simulink model "SC228_TrackedASModelUnitTest"  (R2018b)
settings: Solver=VariableStepAuto  StartTime=0.0  StopTime=10.0  RelTol=1e-3
undefined symbols (not defined in the file or in its folder): ac1dyn_alt0_ft, ac1dyn_con, ac1dyn_lat0_rad, ac1dyn_lon0_rad, ac2dyn_alt0_ft, ac2dyn_con, ac2dyn_lat0_rad, ac2dyn_lon0_rad, ddh_ftps2, dh_ftps, dv_ftps2, e_ft, Edot_ftps, h_ft, hdot_ftps, latLonAltState, n_ft, Ndot_ftps, p_radps, phi_rad, phidot_radps, psi_rad, psidot_radps, q_radps, r_radps, theta_rad, thetadot_radps, uas_tcas_trckd_altQuant_ft, uas_tcas_trckd_bearing_Breakpoints_deg, uas_tcas_trckd_bearing_Max_deg, uas_tcas_trckd_bearing_Sigma_deg, uas_tcas_trckd_dt_s, uas_tcas_trckd_FOR_elev_max_deg, uas_tcas_trckd_FOR_elev_min_deg, uas_tcas_trckd_probDetect, uas_tcas_trckd_psi_bias_ft, uas_tcas_trckd_psi_stddev_ft, uas_tcas_trckd_psidot_bias_radps, uas_tcas_trckd_psidot_stddev_ftps, uas_tcas_trckd_randProbSeed, uas_tcas_trckd_reported_errorCovRBA, uas_tcas_trckd_rng_bias_ft, uas_tcas_trckd_rng_random_stddev_ft, uas_tcas_trckd_seed1, uas_tcas_trckd_seed2, uas_tcas_trckd_seed3, uas_tcas_trckd_seed4, uas_tcas_trckd_sns_max_front_range_ft, uas_tcas_trckd_sns_max_range_ft, uas_tcas_trckd_sns_max_rear_range_ft, uas_tcas_trckd_sns_max_side_range_ft, uas_tcas_trckd_tauThreshold_sec, uas_tcas_trckd_updateRate_sec, v_ftps, vdot_fpss
libraries: simulink x20, dspmtrx3 x1
(part 2 of 2)

== system SC228_TrackedASModelUnitTest/AC2 - Track Following/Follow Trajectory/Set State ==
  x : Inport
  Bus Assignment : BusAssignment  AssignedSignals=v_ftps,n_ft,e_ft,h_ft,psi_rad,theta_rad,phi_rad,dv_ftps2,dh_ftps,ddh_ftps2
  Demux : Demux  Outputs=10
  Null AircraftState : Subsystem
  State : Outport
  wires:
  Demux/10 -> Bus Assignment/11
  Demux/9 -> Bus Assignment/10
  Bus Assignment/1 -> State/1
  Null AircraftState/1(State) -> Bus Assignment/1
  Demux/7 -> Bus Assignment/8  "phi"
  x/1 -> Demux/1
  Demux/6 -> Bus Assignment/7  "theta"
  Demux/5 -> Bus Assignment/6  "psi"
  Demux/4 -> Bus Assignment/5  "h"
  Demux/3 -> Bus Assignment/4  "E"
  Demux/2 -> Bus Assignment/3  "N"
  Demux/1 -> Bus Assignment/2  "v"
  Demux/8 -> Bus Assignment/9  "a"

== system SC228_TrackedASModelUnitTest/SC-228 Sensor Model: Active Surveillance (Tracked)/Add Errors/Colored Noise1 ==
  Add : Sum  Inputs=+++
  Add1 : Sum
  Constant : Constant  Value=false
  Constant1 : Constant  Value=0
  Gain : Gain  Gain=exp(-dt(1)/tau)
  Gain1 : Gain  Gain=sig*sqrt(1-(exp(-dt(1)/tau))*(exp(-dt(1)/tau)))
  Gain2 : Gain  Gain=sig
  IsInitial : Memory  InitialCondition=true  InheritSampleTime=on
  Memory : Memory  InheritSampleTime=on
  Random Number : RandomNumber  Seed=seed  SampleTime=dt_s
  Switch : Switch  Criteria=u2 ~= 0
  bias : Constant  Value=bias
  noisy : Outport
  wires:
  Gain1/1 -> Add1/2  "uncorrelated error"
  Switch/1 -> Memory/1, Add/3  "colored random error"
  bias/1 -> Add/2  "fixed bias"
  Random Number/1 -> Gain2/1, Gain1/1
  Gain/1 -> Add1/1  "correlated error"
  Add/1 -> noisy/1  "noisy state parameter"
  Memory/1 -> Gain/1
  Constant/1 -> IsInitial/1
  IsInitial/1 -> Switch/2
  Add1/1 -> Switch/3  "colored random error"
  Gain2/1 -> Switch/1
  Constant1/1 -> Add/1

== system SC228_TrackedASModelUnitTest/SC-228 Sensor Model: Active Surveillance (Tracked)/Add Errors/Colored Noise2 ==
  Add : Sum  Inputs=+++
  Add1 : Sum
  Constant : Constant  Value=false
  Constant1 : Constant  Value=0
  Gain : Gain  Gain=exp(-dt(1)/tau)
  Gain1 : Gain  Gain=sig*sqrt(1-(exp(-dt(1)/tau))*(exp(-dt(1)/tau)))
  Gain2 : Gain  Gain=sig
  IsInitial : Memory  InitialCondition=true  InheritSampleTime=on
  Memory : Memory  InheritSampleTime=on
  Random Number : RandomNumber  Seed=seed  SampleTime=dt_s
  Switch : Switch  Criteria=u2 ~= 0
  bias : Constant  Value=bias
  noisy : Outport
  wires:
  Gain1/1 -> Add1/2  "uncorrelated error"
  Switch/1 -> Memory/1, Add/3  "colored random error"
  bias/1 -> Add/2  "fixed bias"
  Random Number/1 -> Gain2/1, Gain1/1
  Gain/1 -> Add1/1  "correlated error"
  Add/1 -> noisy/1  "noisy state parameter"
  Memory/1 -> Gain/1
  Constant/1 -> IsInitial/1
  IsInitial/1 -> Switch/2
  Add1/1 -> Switch/3  "colored random error"
  Gain2/1 -> Switch/1
  Constant1/1 -> Add/1

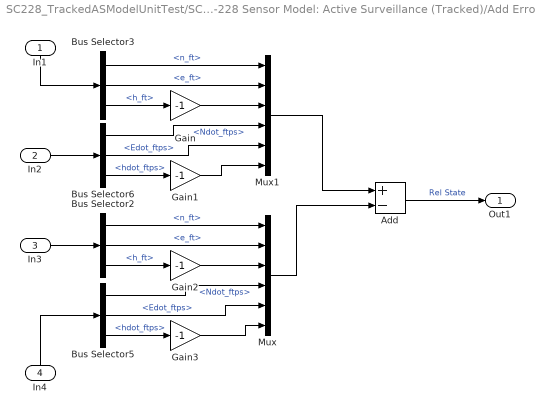
== system SC228_TrackedASModelUnitTest/SC-228 Sensor Model: Active Surveillance (Tracked)/Add Errors/Compute Relative State ==
  In1 : Inport
  In2 : Inport  Port=2
  In3 : Inport  Port=3
  In4 : Inport  Port=4
  Add : Sum  Inputs=+-
  Bus Selector2 : BusSelector  OutputSignals=n_ft,e_ft,h_ft
  Bus Selector3 : BusSelector  OutputSignals=n_ft,e_ft,h_ft
  Bus Selector5 : BusSelector  OutputSignals=Ndot_ftps,Edot_ftps,hdot_ftps
  Bus Selector6 : BusSelector  OutputSignals=Ndot_ftps,Edot_ftps,hdot_ftps
  Gain{,1..3} (4 alike) : Gain  Gain=-1
  Mux : Mux  Inputs=6
  Mux1 : Mux  Inputs=6
  Out1 : Outport
  wires:
  Bus Selector5/1 -> Mux/4  "<Ndot_ftps>"
  Bus Selector5/2 -> Mux/5  "<Edot_ftps>"
  In2/1 -> Bus Selector6/1
  Bus Selector3/3 -> Gain/1  "<h_ft>"
  Bus Selector2/3 -> Gain2/1  "<h_ft>"
  Bus Selector5/3 -> Gain3/1  "<hdot_ftps>"
  Bus Selector2/2 -> Mux/2  "<e_ft>"
  Mux1/1 -> Add/1
  In4/1 -> Bus Selector5/1
  In3/1 -> Bus Selector2/1
  Add/1 -> Out1/1  "Rel State"
  Mux/1 -> Add/2
  Bus Selector2/1 -> Mux/1  "<n_ft>"
  Bus Selector3/1 -> Mux1/1  "<n_ft>"
  Bus Selector3/2 -> Mux1/2  "<e_ft>"
  In1/1 -> Bus Selector3/1
  Bus Selector6/3 -> Gain1/1  "<hdot_ftps>"
  Bus Selector6/1 -> Mux1/4  "<Ndot_ftps>"
  Bus Selector6/2 -> Mux1/5  "<Edot_ftps>"
  Gain/1 -> Mux1/3
  Gain1/1 -> Mux1/6
  Gain2/1 -> Mux/3
  Gain3/1 -> Mux/6

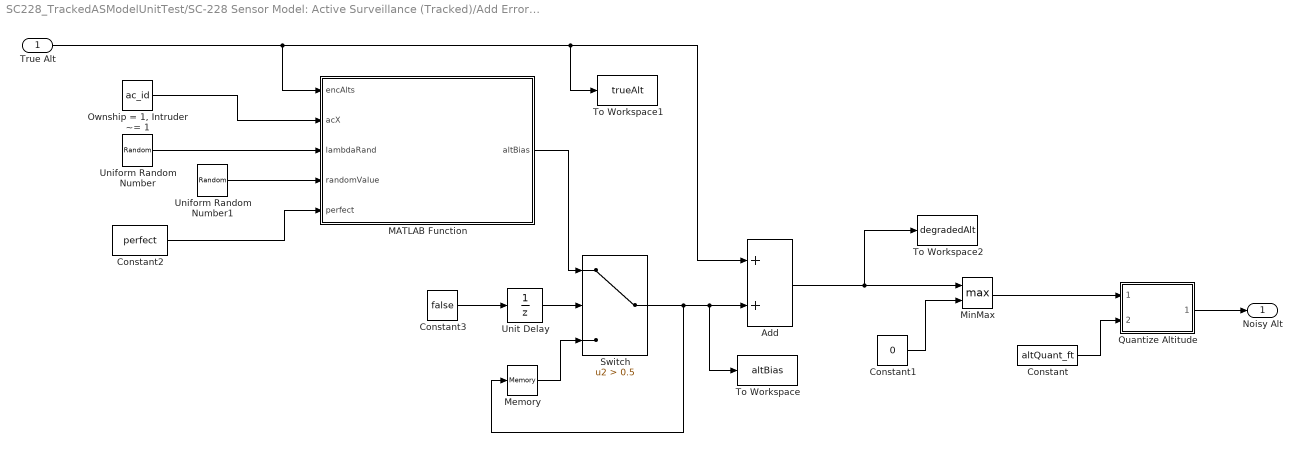
== system SC228_TrackedASModelUnitTest/SC-228 Sensor Model: Active Surveillance (Tracked)/Add Errors/TSAA Altitude Error Model ==
  True Alt : Inport
  Add : Sum
  Constant : Constant  Value=altQuant_ft
  Constant1 : Constant  Value=0
  Constant2 : Constant  Value=perfect
  Constant3 : Constant  Value=false
  MATLAB Function : MATLAB Function  TreatAsAtomicUnit=on
  Memory : Memory
  MinMax : MinMax  Function=max  Inputs=2
  "Ownship = 1, Intruder ~= 1" : Constant  Value=ac_id
  Quantize Altitude : Subsystem
  Switch : Switch  Criteria=u2 > Threshold  Threshold=0.5
  To Workspace : ToWorkspace  VariableName=altBias  SaveFormat=Timeseries  SampleTime=-1
  To Workspace1 : ToWorkspace  VariableName=trueAlt  SaveFormat=Timeseries  SampleTime=-1
  To Workspace2 : ToWorkspace  VariableName=degradedAlt  SaveFormat=Timeseries  SampleTime=-1
  Uniform Random Number : UniformRandomNumber  Minimum=0  Seed=lambdaSeed  SampleTime=dt_s
  Uniform Random Number1 : UniformRandomNumber  Minimum=0  Seed=randomSeed  SampleTime=dt_s
  Unit Delay : UnitDelay  InitialCondition=true  SampleTime=-1
  Noisy Alt : Outport
  wires:
  Constant2/1 -> MATLAB Function/5(perfect)
  Quantize Altitude/1(Quantized Alt) -> Noisy Alt/1
  MinMax/1 -> Quantize Altitude/1(Altitude)
  Constant1/1 -> MinMax/2
  "Ownship = 1, Intruder ~= 1"/1 -> MATLAB Function/2(acX)
  True Alt/1 -> To Workspace1/1, Add/1, MATLAB Function/1(encAlts)
  Uniform Random Number/1 -> MATLAB Function/3(lambdaRand)
  Uniform Random Number1/1 -> MATLAB Function/4(randomValue)
  MATLAB Function/1(altBias) -> Switch/1
  Constant3/1 -> Unit Delay/1
  Unit Delay/1 -> Switch/2
  Switch/1 -> To Workspace/1, Add/2, Memory/1
  Memory/1 -> Switch/3
  Constant/1 -> Quantize Altitude/2(Quant_level)
  Add/1 -> To Workspace2/1, MinMax/1

== system SC228_TrackedASModelUnitTest/SC-228 Sensor Model: Active Surveillance (Tracked)/Add Errors/White Noise ==
  bearing : Inport
  MATLAB Function : MATLAB Function  TreatAsAtomicUnit=on
  Random Number : RandomNumber  Seed=seed_bearing  SampleTime=dt_s
  Terminator : Terminator
  To Workspace : ToWorkspace  VariableName=psi  SaveFormat=Timeseries  SampleTime=-1
  "noisy " : Outport
  psiSigma : Outport  Port=2
  wires:
  MATLAB Function/1(sigma) -> psiSigma/1
  MATLAB Function/2(max) -> Terminator/1
  bearing/1 -> [psi]
  [psi] -> To Workspace/1, "noisy "/1, MATLAB Function/1(psi)

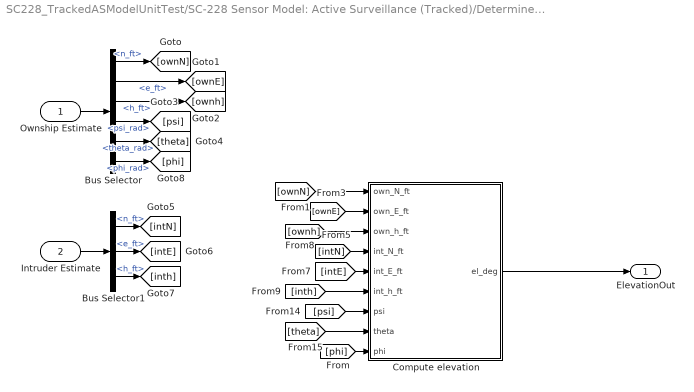
== system SC228_TrackedASModelUnitTest/SC-228 Sensor Model: Active Surveillance (Tracked)/Determine Track Validity/Compute Elevation ==
  Ownship Estimate : Inport
  Intruder Estimate : Inport  Port=2
  Bus Selector : BusSelector  OutputSignals=n_ft,e_ft,h_ft,psi_rad,theta_rad,phi_rad
  Bus Selector1 : BusSelector  OutputSignals=n_ft,e_ft,h_ft
  Compute elevation : MATLAB Function  TreatAsAtomicUnit=on
  ElevationOut : Outport
  wires:
  Ownship Estimate/1 -> Bus Selector/1
  Compute elevation/1(el_deg) -> ElevationOut/1
  Intruder Estimate/1 -> Bus Selector1/1
  Bus Selector/1 -> [ownN]  "<n_ft>"
  Bus Selector/2 -> [ownE]  "<e_ft>"
  Bus Selector/3 -> [ownh]  "<h_ft>"
  Bus Selector/4 -> [psi]  "<psi_rad>"
  Bus Selector/5 -> [theta]  "<theta_rad>"
  Bus Selector1/1 -> [intN]  "<n_ft>"
  Bus Selector1/2 -> [intE]  "<e_ft>"
  Bus Selector1/3 -> [inth]  "<h_ft>"
  [ownN] -> Compute elevation/1(own_N_ft)
  [ownE] -> Compute elevation/2(own_E_ft)
  [intN] -> Compute elevation/4(int_N_ft)
  [intE] -> Compute elevation/5(int_E_ft)
  [ownh] -> Compute elevation/3(own_h_ft)
  [inth] -> Compute elevation/6(int_h_ft)
  [psi] -> Compute elevation/7(psi)
  [theta] -> Compute elevation/8(theta)
  Bus Selector/6 -> [phi]  "<phi_rad>"
  [phi] -> Compute elevation/9(phi)

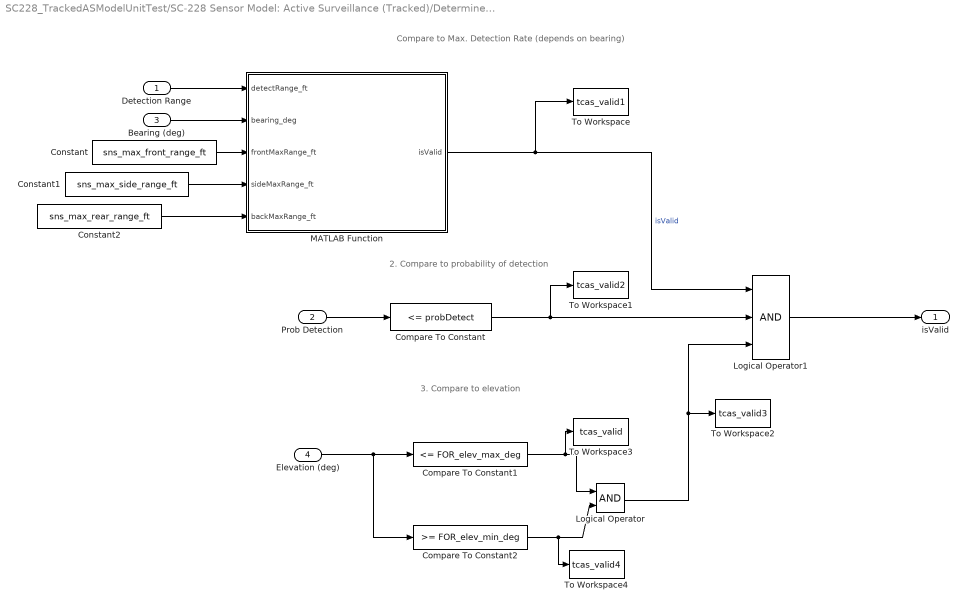
== system SC228_TrackedASModelUnitTest/SC-228 Sensor Model: Active Surveillance (Tracked)/Determine Track Validity/Determine Validity  ==
  note: 3. Compare to elevation
  note: 2. Compare to probability of detection
  note: Compare to Max. Detection Rate (depends on bearing)
  Detection Range : Inport
  Prob Detection : Inport  Port=2
  Bearing (deg) : Inport  Port=3
  Elevation (deg) : Inport  Port=4
  Compare To Constant : simulink/Logic and Bit Operations/Compare To Constant  relop=<=  const=probDetect  OutDataTypeStr=boolean
  Compare To Constant1 : simulink/Logic and Bit Operations/Compare To Constant  relop=<=  const=FOR_elev_max_deg  OutDataTypeStr=boolean
  Compare To Constant2 : simulink/Logic and Bit Operations/Compare To Constant  relop=>=  const=FOR_elev_min_deg  OutDataTypeStr=boolean
  Constant : Constant  Value=sns_max_front_range_ft
  Constant1 : Constant  Value=sns_max_side_range_ft
  Constant2 : Constant  Value=sns_max_rear_range_ft
  Logical Operator : Logic  AllPortsSameDT=off  OutDataTypeStr=boolean
  Logical Operator1 : Logic  Inputs=3  AllPortsSameDT=off  OutDataTypeStr=boolean
  MATLAB Function : MATLAB Function  TreatAsAtomicUnit=on
  To Workspace : ToWorkspace  VariableName=tcas_valid1  SaveFormat=Timeseries  SampleTime=-1
  To Workspace1 : ToWorkspace  VariableName=tcas_valid2  SaveFormat=Timeseries  SampleTime=-1
  To Workspace2 : ToWorkspace  VariableName=tcas_valid3  SaveFormat=Timeseries  SampleTime=-1
  To Workspace3 : ToWorkspace  VariableName=tcas_valid  SaveFormat=Timeseries  SampleTime=-1
  To Workspace4 : ToWorkspace  VariableName=tcas_valid4  SaveFormat=Timeseries  SampleTime=-1
  isValid : Outport
  wires:
  Detection Range/1 -> MATLAB Function/1(detectRange_ft)
  MATLAB Function/1(isValid) -> Logical Operator1/1, To Workspace/1  "isValid"
  Prob Detection/1 -> Compare To Constant/1
  Compare To Constant/1 -> Logical Operator1/2, To Workspace1/1
  Elevation (deg)/1 -> Compare To Constant2/1, Compare To Constant1/1
  Compare To Constant1/1 -> Logical Operator/1, To Workspace3/1
  Compare To Constant2/1 -> Logical Operator/2, To Workspace4/1
  Logical Operator1/1 -> isValid/1
  Logical Operator/1 -> Logical Operator1/3, To Workspace2/1
  Bearing (deg)/1 -> MATLAB Function/2(bearing_deg)
  Constant/1 -> MATLAB Function/3(frontMaxRange_ft)
  Constant1/1 -> MATLAB Function/4(sideMaxRange_ft)
  Constant2/1 -> MATLAB Function/5(backMaxRange_ft)

== system SC228_TrackedASModelUnitTest/AC1 - Track Following/Follow Trajectory/Compute Body Rates/Compute p ==
  State : Inport
  Euler Rates : Inport  Port=2
  Add : Sum
  Bus Selector : BusSelector  OutputSignals=theta_rad
  Bus Selector1 : BusSelector  OutputSignals=psidot,phidot
  Product : Product
  Trigonometric Function : Trigonometry
  Unary Minus : UnaryMinus
  p : Outport
  wires:
  Add/1 -> p/1
  Unary Minus/1 -> Product/1
  Bus Selector1/2 -> Add/2  "<phidot>"
  Product/1 -> Add/1
  Trigonometric Function/1 -> Unary Minus/1
  State/1 -> Bus Selector/1
  Euler Rates/1 -> Bus Selector1/1
  Bus Selector/1 -> Trigonometric Function/1  "<theta_rad>"
  Bus Selector1/1 -> Product/2  "<psidot>"

== system SC228_TrackedASModelUnitTest/AC1 - Track Following/Follow Trajectory/Compute Body Rates/Compute q ==
  State : Inport
  Euler Rates : Inport  Port=2
  Add : Sum
  Bus Selector : BusSelector  OutputSignals=phi_rad,theta_rad
  Bus Selector1 : BusSelector  OutputSignals=thetadot,psidot
  Product : Product
  Product1 : Product  Inputs=3
  Trigonometric Function : Trigonometry  Operator=cos
  Trigonometric Function1 : Trigonometry  Operator=cos
  Trigonometric Function2 : Trigonometry
  q : Outport
  wires:
  Add/1 -> q/1
  Product1/1 -> Add/2
  Bus Selector1/2 -> Product1/3  "<psidot>"
  Trigonometric Function1/1 -> Product1/2
  Trigonometric Function2/1 -> Product1/1
  Bus Selector/2 -> Trigonometric Function1/1  "<theta_rad>"
  Bus Selector1/1 -> Product/2  "<thetadot>"
  Bus Selector/1 -> Trigonometric Function/1, Trigonometric Function2/1  "<phi_rad>"
  Trigonometric Function/1 -> Product/1
  Product/1 -> Add/1
  State/1 -> Bus Selector/1
  Euler Rates/1 -> Bus Selector1/1

== system SC228_TrackedASModelUnitTest/AC1 - Track Following/Follow Trajectory/Compute Body Rates/Compute r ==
  State : Inport
  Euler Rates : Inport  Port=2
  Add : Sum
  Bus Selector : BusSelector  OutputSignals=phi_rad,theta_rad
  Bus Selector1 : BusSelector  OutputSignals=thetadot,psidot
  Product : Product
  Product1 : Product  Inputs=3
  Trigonometric Function : Trigonometry
  Trigonometric Function1 : Trigonometry  Operator=cos
  Trigonometric Function2 : Trigonometry  Operator=cos
  Unary Minus : UnaryMinus
  r : Outport
  wires:
  Unary Minus/1 -> Product/1
  Add/1 -> r/1
  Product1/1 -> Add/2
  Bus Selector1/2 -> Product1/3  "<psidot>"
  Trigonometric Function1/1 -> Product1/2
  Trigonometric Function2/1 -> Product1/1
  Bus Selector/2 -> Trigonometric Function1/1  "<theta_rad>"
  Bus Selector1/1 -> Product/2  "<thetadot>"
  Bus Selector/1 -> Trigonometric Function/1, Trigonometric Function2/1  "<phi_rad>"
  Trigonometric Function/1 -> Unary Minus/1
  Product/1 -> Add/1
  State/1 -> Bus Selector/1
  Euler Rates/1 -> Bus Selector1/1

== system SC228_TrackedASModelUnitTest/AC1 - Track Following/Follow Trajectory/Get Trajectory Data/Compute Accel ==
  speed : Inport
  Discrete Derivative : simulink/Discrete/Discrete Derivative  gainval=1.0  ICPrevScaledInput=0.0  OutMin=[]  OutMax=[]  OutDataType=fixdt(1, 16)  OutScaling=2^-10  DoSatur=off
  accel : Outport
  wires:
  Discrete Derivative/1 -> accel/1
  speed/1 -> Discrete Derivative/1

== system SC228_TrackedASModelUnitTest/AC1 - Track Following/Follow Trajectory/Get Trajectory Data/Compute Accel1 ==
  speed : Inport
  Discrete Derivative : simulink/Discrete/Discrete Derivative  gainval=1.0  ICPrevScaledInput=0.0  OutMin=[]  OutMax=[]  OutDataType=fixdt(1, 16)  OutScaling=2^-10  DoSatur=off
  accel : Outport
  wires:
  Discrete Derivative/1 -> accel/1
  speed/1 -> Discrete Derivative/1

== system SC228_TrackedASModelUnitTest/AC1 - Track Following/Follow Trajectory/Get Trajectory Data/Compute Bank Angle ==
  speed : Inport
  psi : Inport  Port=2
  Constant : Constant  Value=32.2
  Discrete Derivative : simulink/Discrete/Discrete Derivative  gainval=1.0  ICPrevScaledInput=0.0  OutMin=[]  OutMax=[]  OutDataType=fixdt(1, 16)  OutScaling=2^-10  DoSatur=off
  Divide : Product  Inputs=*/
  IC : InitialCondition  Value=0
  Product : Product
  Trigonometric Function : Trigonometry  Operator=atan
  phi : Outport
  wires:
  IC/1 -> Product/2
  Trigonometric Function/1 -> phi/1
  Divide/1 -> Trigonometric Function/1
  Constant/1 -> Divide/2
  Product/1 -> Divide/1
  psi/1 -> Discrete Derivative/1  "psi"
  speed/1 -> Product/1  "speed"
  Discrete Derivative/1 -> IC/1  "psidot"

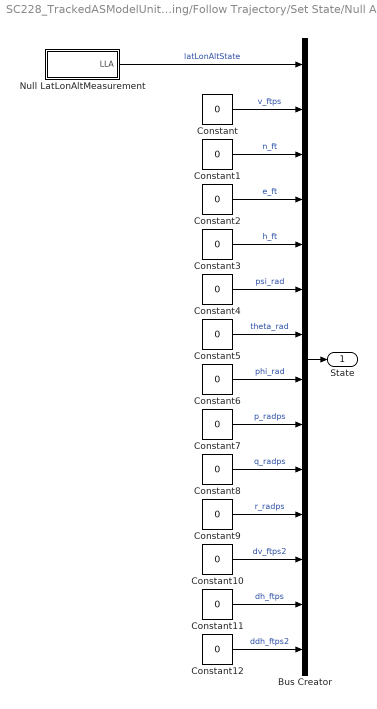
== system SC228_TrackedASModelUnitTest/AC1 - Track Following/Follow Trajectory/Set State/Null AircraftState ==
  Bus Creator : BusCreator  Inputs='latLonAltState','v_ftps','n_ft','e_ft','h_ft','psi_rad','theta_rad','phi_rad','p_radps','q_radps','r_radps','dv_ftps2','dh_ftps','ddh_ftps2'  OutDataTypeStr=Bus: AircraftState
  Constant{,1..12} (13 alike) : Constant  Value=0
  Null LatLonAltMeasurement : Subsystem
  State : Outport
  wires:
  Null LatLonAltMeasurement/1(LLA) -> Bus Creator/1  "latLonAltState"
  Constant/1 -> Bus Creator/2  "v_ftps"
  Constant12/1 -> Bus Creator/14  "ddh_ftps2"
  Constant1/1 -> Bus Creator/3  "n_ft"
  Bus Creator/1 -> State/1
  Constant6/1 -> Bus Creator/8  "phi_rad"
  Constant10/1 -> Bus Creator/12  "dv_ftps2"
  Constant7/1 -> Bus Creator/9  "p_radps"
  Constant5/1 -> Bus Creator/7  "theta_rad"
  Constant4/1 -> Bus Creator/6  "psi_rad"
  Constant8/1 -> Bus Creator/10  "q_radps"
  Constant9/1 -> Bus Creator/11  "r_radps"
  Constant3/1 -> Bus Creator/5  "h_ft"
  Constant2/1 -> Bus Creator/4  "e_ft"
  Constant11/1 -> Bus Creator/13  "dh_ftps"

== system SC228_TrackedASModelUnitTest/AC2 - Track Following/Follow Trajectory/Compute Body Rates/Compute p ==
  State : Inport
  Euler Rates : Inport  Port=2
  Add : Sum
  Bus Selector : BusSelector  OutputSignals=theta_rad
  Bus Selector1 : BusSelector  OutputSignals=psidot,phidot
  Product : Product
  Trigonometric Function : Trigonometry
  Unary Minus : UnaryMinus
  p : Outport
  wires:
  Add/1 -> p/1
  Unary Minus/1 -> Product/1
  Bus Selector1/2 -> Add/2  "<phidot>"
  Product/1 -> Add/1
  Trigonometric Function/1 -> Unary Minus/1
  State/1 -> Bus Selector/1
  Euler Rates/1 -> Bus Selector1/1
  Bus Selector/1 -> Trigonometric Function/1  "<theta_rad>"
  Bus Selector1/1 -> Product/2  "<psidot>"

== system SC228_TrackedASModelUnitTest/AC2 - Track Following/Follow Trajectory/Compute Body Rates/Compute q ==
  State : Inport
  Euler Rates : Inport  Port=2
  Add : Sum
  Bus Selector : BusSelector  OutputSignals=phi_rad,theta_rad
  Bus Selector1 : BusSelector  OutputSignals=thetadot,psidot
  Product : Product
  Product1 : Product  Inputs=3
  Trigonometric Function : Trigonometry  Operator=cos
  Trigonometric Function1 : Trigonometry  Operator=cos
  Trigonometric Function2 : Trigonometry
  q : Outport
  wires:
  Add/1 -> q/1
  Product1/1 -> Add/2
  Bus Selector1/2 -> Product1/3  "<psidot>"
  Trigonometric Function1/1 -> Product1/2
  Trigonometric Function2/1 -> Product1/1
  Bus Selector/2 -> Trigonometric Function1/1  "<theta_rad>"
  Bus Selector1/1 -> Product/2  "<thetadot>"
  Bus Selector/1 -> Trigonometric Function/1, Trigonometric Function2/1  "<phi_rad>"
  Trigonometric Function/1 -> Product/1
  Product/1 -> Add/1
  State/1 -> Bus Selector/1
  Euler Rates/1 -> Bus Selector1/1

== system SC228_TrackedASModelUnitTest/AC2 - Track Following/Follow Trajectory/Compute Body Rates/Compute r ==
  State : Inport
  Euler Rates : Inport  Port=2
  Add : Sum
  Bus Selector : BusSelector  OutputSignals=phi_rad,theta_rad
  Bus Selector1 : BusSelector  OutputSignals=thetadot,psidot
  Product : Product
  Product1 : Product  Inputs=3
  Trigonometric Function : Trigonometry
  Trigonometric Function1 : Trigonometry  Operator=cos
  Trigonometric Function2 : Trigonometry  Operator=cos
  Unary Minus : UnaryMinus
  r : Outport
  wires:
  Unary Minus/1 -> Product/1
  Add/1 -> r/1
  Product1/1 -> Add/2
  Bus Selector1/2 -> Product1/3  "<psidot>"
  Trigonometric Function1/1 -> Product1/2
  Trigonometric Function2/1 -> Product1/1
  Bus Selector/2 -> Trigonometric Function1/1  "<theta_rad>"
  Bus Selector1/1 -> Product/2  "<thetadot>"
  Bus Selector/1 -> Trigonometric Function/1, Trigonometric Function2/1  "<phi_rad>"
  Trigonometric Function/1 -> Unary Minus/1
  Product/1 -> Add/1
  State/1 -> Bus Selector/1
  Euler Rates/1 -> Bus Selector1/1

== system SC228_TrackedASModelUnitTest/AC2 - Track Following/Follow Trajectory/Get Trajectory Data/Compute Accel ==
  speed : Inport
  Discrete Derivative : simulink/Discrete/Discrete Derivative  gainval=1.0  ICPrevScaledInput=0.0  OutMin=[]  OutMax=[]  OutDataType=fixdt(1, 16)  OutScaling=2^-10  DoSatur=off
  accel : Outport
  wires:
  Discrete Derivative/1 -> accel/1
  speed/1 -> Discrete Derivative/1

== system SC228_TrackedASModelUnitTest/AC2 - Track Following/Follow Trajectory/Get Trajectory Data/Compute Accel1 ==
  speed : Inport
  Discrete Derivative : simulink/Discrete/Discrete Derivative  gainval=1.0  ICPrevScaledInput=0.0  OutMin=[]  OutMax=[]  OutDataType=fixdt(1, 16)  OutScaling=2^-10  DoSatur=off
  accel : Outport
  wires:
  Discrete Derivative/1 -> accel/1
  speed/1 -> Discrete Derivative/1

== system SC228_TrackedASModelUnitTest/AC2 - Track Following/Follow Trajectory/Get Trajectory Data/Compute Bank Angle ==
  speed : Inport
  psi : Inport  Port=2
  Constant : Constant  Value=32.2
  Discrete Derivative : simulink/Discrete/Discrete Derivative  gainval=1.0  ICPrevScaledInput=0.0  OutMin=[]  OutMax=[]  OutDataType=fixdt(1, 16)  OutScaling=2^-10  DoSatur=off
  Divide : Product  Inputs=*/
  IC : InitialCondition  Value=0
  Product : Product
  Trigonometric Function : Trigonometry  Operator=atan
  phi : Outport
  wires:
  IC/1 -> Product/2
  Trigonometric Function/1 -> phi/1
  Divide/1 -> Trigonometric Function/1
  Constant/1 -> Divide/2
  Product/1 -> Divide/1
  psi/1 -> Discrete Derivative/1  "psi"
  speed/1 -> Product/1  "speed"
  Discrete Derivative/1 -> IC/1  "psidot"

== system SC228_TrackedASModelUnitTest/AC2 - Track Following/Follow Trajectory/Set State/Null AircraftState ==
  Bus Creator : BusCreator  Inputs='latLonAltState','v_ftps','n_ft','e_ft','h_ft','psi_rad','theta_rad','phi_rad','p_radps','q_radps','r_radps','dv_ftps2','dh_ftps','ddh_ftps2'  OutDataTypeStr=Bus: AircraftState
  Constant{,1..12} (13 alike) : Constant  Value=0
  Null LatLonAltMeasurement : Subsystem
  State : Outport
  wires:
  Null LatLonAltMeasurement/1(LLA) -> Bus Creator/1  "latLonAltState"
  Constant/1 -> Bus Creator/2  "v_ftps"
  Constant12/1 -> Bus Creator/14  "ddh_ftps2"
  Constant1/1 -> Bus Creator/3  "n_ft"
  Bus Creator/1 -> State/1
  Constant6/1 -> Bus Creator/8  "phi_rad"
  Constant10/1 -> Bus Creator/12  "dv_ftps2"
  Constant7/1 -> Bus Creator/9  "p_radps"
  Constant5/1 -> Bus Creator/7  "theta_rad"
  Constant4/1 -> Bus Creator/6  "psi_rad"
  Constant8/1 -> Bus Creator/10  "q_radps"
  Constant9/1 -> Bus Creator/11  "r_radps"
  Constant3/1 -> Bus Creator/5  "h_ft"
  Constant2/1 -> Bus Creator/4  "e_ft"
  Constant11/1 -> Bus Creator/13  "dh_ftps"

== system SC228_TrackedASModelUnitTest/SC-228 Sensor Model: Active Surveillance (Tracked)/Add Errors/TSAA Altitude Error Model/Quantize Altitude ==
  note: quant_level * round(alt/quant_level)
  Altitude : Inport
  Quant_level : Inport  Port=2
  Divide : Product  Inputs=*/
  Product : Product
  Rounding Function : Rounding  Operator=round
  Quantized Alt : Outport
  wires:
  Altitude/1 -> Divide/1
  Quant_level/1 -> Product/2, Divide/2
  Divide/1 -> Rounding Function/1
  Rounding Function/1 -> Product/1
  Product/1 -> Quantized Alt/1

== system SC228_TrackedASModelUnitTest/AC1 - Track Following/Follow Trajectory/Set State/Null AircraftState/Null LatLonAltMeasurement ==
  Bus Creator : BusCreator  Inputs='lat_rad','lon_rad','dlat_radps','dlon_radps','alt_ft','dalt_ftps'  OutDataTypeStr=Bus: LatLonAltMeasurement
  Constant{,1..5} (6 alike) : Constant  Value=0
  LLA : Outport
  wires:
  Constant1/1 -> Bus Creator/2  "lon_rad"
  Bus Creator/1 -> LLA/1
  Constant4/1 -> Bus Creator/5  "alt_ft"
  Constant5/1 -> Bus Creator/6  "dalt_ftps"
  Constant3/1 -> Bus Creator/4  "dlon_radps"
  Constant/1 -> Bus Creator/1  "lat_rad"
  Constant2/1 -> Bus Creator/3  "dlat_radps"

== system SC228_TrackedASModelUnitTest/AC2 - Track Following/Follow Trajectory/Set State/Null AircraftState/Null LatLonAltMeasurement ==
  Bus Creator : BusCreator  Inputs='lat_rad','lon_rad','dlat_radps','dlon_radps','alt_ft','dalt_ftps'  OutDataTypeStr=Bus: LatLonAltMeasurement
  Constant{,1..5} (6 alike) : Constant  Value=0
  LLA : Outport
  wires:
  Constant1/1 -> Bus Creator/2  "lon_rad"
  Bus Creator/1 -> LLA/1
  Constant4/1 -> Bus Creator/5  "alt_ft"
  Constant5/1 -> Bus Creator/6  "dalt_ftps"
  Constant3/1 -> Bus Creator/4  "dlon_radps"
  Constant/1 -> Bus Creator/1  "lat_rad"
  Constant2/1 -> Bus Creator/3  "dlat_radps"

== matlab function SC228_TrackedASModelUnitTest/AC1 - Track Following/Follow Trajectory/Set LLA /MATLAB Function ==
  data: e_ft input; n_ft input; u_ft input; v_ftps input; psi_rad input; theta_rad input; lat0 input; lat_rad output; lon0 input; h0 input; lon_rad output; dlat_radps output; dlon_radps output; alt_ft output; dalt_ftps output
function [lat_rad,lon_rad,dlat_radps,dlon_radps,alt_ft,dalt_ftps] = convertToLLA(e_ft,n_ft,u_ft,v_ftps,psi_rad,theta_rad,lat0,lon0,h0)
%#codegen

% WGS-84 ellipsoid constants
a = 2.09256*10^7;          %Semi-major axis (meters)
f = 1.0/298.257223563;  %Flattening
ecc_sq = f*(2.0-f);        %Eccentricity^2


% Ellipsoidal "radius"
er = a./sqrt(1-ecc_sq.*sin(lat0).^2);


% ECEF coordinates
x0 = (er + h0)*cos(lat0)*cos(lon0);
y0 = (er + h0)*cos(lat0)*sin(lon0);
z0 = (er.*(1-ecc_sq) + h0)*sin(lat0);


%% Rotation Matrix
posECEF0 = [x0;y0;z0];
% Compute the local Up unit vector
vHatU = posECEF0;
vHatU(3) = vHatU(3) ./ ((1-f)^2);
vHatU = vHatU ./ norm(vHatU);

% Compute the projection onto the local Up vector
pU = vHatU * vHatU';

% Compute the projection onto the local Tangent plane
pT = eye(size(pU)) - pU;

% Compute the local North unit vector
vHatZ = [0;0;1];
vHatN = pT * vHatZ;
vHatN = vHatN ./ norm(vHatN);

% Compute the local East unit vector
vHatE = cross(vHatN,vHatU);

% Compute ENU rotation matrix
rotMatENU = zeros(3,3);
rotMatENU(:,1) = vHatE;
rotMatENU(:,2) = vHatN;
rotMatENU(:,3) = vHatU;

tPosECEF = rotMatENU*[e_ft;n_ft;u_ft] + [x0;y0;z0];


%% ECEF to LLA
% WGS-84 derived parameters
b = (1-f).*a;                       %Semi-minor axis (meters)
ecc1_sq = (a.^2 - b.^2)./(a.^2);    %First eccentricity squared
ecc2_sq = (a.^2 - b.^2)./(b.^2);    %Second eccentricity squared


% Length of position vector in equatorial plane
rho = sqrt(tPosECEF(1).^2 + tPosECEF(2).^2);

% Auxillary angle
theta = atan( (tPosECEF(3).*a)./(rho.*b) );

lon_rad = atan2(tPosECEF(2),tPosECEF(1));
lat_rad = atan( (tPosECEF(3) + ecc2_sq.*b.*(sin(theta)).^3)./(rho - ecc1_sq.*a.*(cos(theta)).^3) );

ewRadCurv = a./sqrt(1-ecc1_sq.*sin(lat_rad).^2);

alt_ft = (rho./cos(lat_rad)) - ewRadCurv;


%% Velocities - Project 1 sec into future and use to estimate
dalt_ftps = v_ftps*sin(theta_rad); % Assume about the same


tPosECEF_1sec = rotMatENU*[e_ft+v_ftps*sin(theta_rad)*sin(psi_rad);...
                           n_ft+v_ftps*sin(theta_rad)*cos(psi_rad);...
                           u_ft] + ...
                           [x0;y0;z0];

% Length of position vector in equatorial plane
rho = sqrt(tPosECEF_1sec(1).^2 + tPosECEF_1sec(2).^2);

% Auxillary angle
theta = atan( (tPosECEF_1sec(3).*a)./(rho.*b) );

lon_rad_1sec = atan2(tPosECEF_1sec(2),tPosECEF_1sec(1));
lat_rad_1sec = atan( (tPosECEF_1sec(3) + ecc2_sq.*b.*(sin(theta)).^3)./(rho - ecc1_sq.*a.*(cos(theta)).^3) );

dlat_radps = lat_rad_1sec - lat_rad;
dlon_radps = lon_rad_1sec - lon_rad;
end

== matlab function SC228_TrackedASModelUnitTest/AC2 - Track Following/Follow Trajectory/Set LLA /MATLAB Function ==
  data: e_ft input; n_ft input; u_ft input; v_ftps input; psi_rad input; theta_rad input; lat0 input; lat_rad output; lon0 input; h0 input; lon_rad output; dlat_radps output; dlon_radps output; alt_ft output; dalt_ftps output
function [lat_rad,lon_rad,dlat_radps,dlon_radps,alt_ft,dalt_ftps] = convertToLLA(e_ft,n_ft,u_ft,v_ftps,psi_rad,theta_rad,lat0,lon0,h0)
%#codegen

% WGS-84 ellipsoid constants
a = 2.09256*10^7;          %Semi-major axis (meters)
f = 1.0/298.257223563;  %Flattening
ecc_sq = f*(2.0-f);        %Eccentricity^2


% Ellipsoidal "radius"
er = a./sqrt(1-ecc_sq.*sin(lat0).^2);


% ECEF coordinates
x0 = (er + h0)*cos(lat0)*cos(lon0);
y0 = (er + h0)*cos(lat0)*sin(lon0);
z0 = (er.*(1-ecc_sq) + h0)*sin(lat0);


%% Rotation Matrix
posECEF0 = [x0;y0;z0];
% Compute the local Up unit vector
vHatU = posECEF0;
vHatU(3) = vHatU(3) ./ ((1-f)^2);
vHatU = vHatU ./ norm(vHatU);

% Compute the projection onto the local Up vector
pU = vHatU * vHatU';

% Compute the projection onto the local Tangent plane
pT = eye(size(pU)) - pU;

% Compute the local North unit vector
vHatZ = [0;0;1];
vHatN = pT * vHatZ;
vHatN = vHatN ./ norm(vHatN);

% Compute the local East unit vector
vHatE = cross(vHatN,vHatU);

% Compute ENU rotation matrix
rotMatENU = zeros(3,3);
rotMatENU(:,1) = vHatE;
rotMatENU(:,2) = vHatN;
rotMatENU(:,3) = vHatU;

tPosECEF = rotMatENU*[e_ft;n_ft;u_ft] + [x0;y0;z0];


%% ECEF to LLA
% WGS-84 derived parameters
b = (1-f).*a;                       %Semi-minor axis (meters)
ecc1_sq = (a.^2 - b.^2)./(a.^2);    %First eccentricity squared
ecc2_sq = (a.^2 - b.^2)./(b.^2);    %Second eccentricity squared


% Length of position vector in equatorial plane
rho = sqrt(tPosECEF(1).^2 + tPosECEF(2).^2);

% Auxillary angle
theta = atan( (tPosECEF(3).*a)./(rho.*b) );

lon_rad = atan2(tPosECEF(2),tPosECEF(1));
lat_rad = atan( (tPosECEF(3) + ecc2_sq.*b.*(sin(theta)).^3)./(rho - ecc1_sq.*a.*(cos(theta)).^3) );

ewRadCurv = a./sqrt(1-ecc1_sq.*sin(lat_rad).^2);

alt_ft = (rho./cos(lat_rad)) - ewRadCurv;


%% Velocities - Project 1 sec into future and use to estimate
dalt_ftps = v_ftps*sin(theta_rad); % Assume about the same


tPosECEF_1sec = rotMatENU*[e_ft+v_ftps*sin(theta_rad)*sin(psi_rad);...
                           n_ft+v_ftps*sin(theta_rad)*cos(psi_rad);...
                           u_ft] + ...
                           [x0;y0;z0];

% Length of position vector in equatorial plane
rho = sqrt(tPosECEF_1sec(1).^2 + tPosECEF_1sec(2).^2);

% Auxillary angle
theta = atan( (tPosECEF_1sec(3).*a)./(rho.*b) );

lon_rad_1sec = atan2(tPosECEF_1sec(2),tPosECEF_1sec(1));
lat_rad_1sec = atan( (tPosECEF_1sec(3) + ecc2_sq.*b.*(sin(theta)).^3)./(rho - ecc1_sq.*a.*(cos(theta)).^3) );

dlat_radps = lat_rad_1sec - lat_rad;
dlon_radps = lon_rad_1sec - lon_rad;
end

== matlab function SC228_TrackedASModelUnitTest/SC-228 Sensor Model: Active Surveillance (Tracked)/Add Errors/TSAA Altitude Error Model/MATLAB Function ==
  data: encAlts input; altBias output; acX input; lambdaRand input; randomValue input; perfect input
function altBias  = degradeAlt(encAlts, acX, lambdaRand, randomValue, perfect)

altBias = TSAA_Model_External_Functions.degradeAlt(encAlts, acX, lambdaRand, randomValue, perfect);

== matlab function SC228_TrackedASModelUnitTest/SC-228 Sensor Model: Active Surveillance (Tracked)/Add Errors/White Noise/MATLAB Function ==
  data: psi input; sigma output; max output
function [sigma, max]= fcn(psi)
%#codegen
sigma = 0; max = 0;

bearing_Breakpoints_deg = [-9999, -15, -10, 10, 20, 9999]';
bearing_Sigma_deg = [15, 15, 15, 9, 15, 15];
bearing_Max_deg = [45, 45, 45, 27, 45, 45];

index = find(psi<bearing_Breakpoints_deg,1);
index = index(1);

sigma = bearing_Sigma_deg(index);
max = bearing_Max_deg(index);

== matlab function SC228_TrackedASModelUnitTest/SC-228 Sensor Model: Active Surveillance (Tracked)/Add Errors/xyz2cyl ==
  data: xRel input; r output; yRel input; zRel input; xDotRel input; yDotRel input; zDotRel input; ownPsi input; ownPsiDot input; rDot output; b output; bDot output; h output; hDot output; J output; K output
function [r,rDot,b,bDot,h,hDot,J,K] = fcn(xRel,yRel,zRel,xDotRel,yDotRel,zDotRel,ownPsi,ownPsiDot)
%#codegen
% Convert position and velocity of intruder relative to ownship from 
% Cartesian coordinates in North-East-Down system to range/bearing/altitude
% coordinates.  Also returns Jacobian blocks J and K, where 6x6 Jacobian =
% [J zeros; K J]

r = norm([xRel yRel zRel]);
h = -zRel;
b = atan2(yRel,xRel) - ownPsi;

rDot = dot([xRel yRel zRel], [xDotRel yDotRel zDotRel])/r;
hDot = -zDotRel;
bDot = (yDotRel*xRel - yRel*xDotRel)/(xRel^2 + yRel^2) - ownPsiDot;

r2D = norm([xRel yRel]);

% Jacobian elements

J = [  xRel/r   yRel/r   zRel/r ;
     -yRel/r2D^2 xRel/r2D^2    0    ;
          0       0       -1   ];
      
K = zeros(3,3);
K(1,1) = xDotRel/r - xRel*rDot/r^2;
K(1,2) = yDotRel/r - yRel*rDot/r^2;
K(1,3) = zDotRel/r - zRel*rDot/r^2;
K(2,1) = (yDotRel*yRel^2 + 2*xRel*xDotRel*yRel - yDotRel*xRel^2)/r2D^4;
K(2,2) = (xDotRel*yRel^2 - 2*xRel*yRel*yDotRel - xRel^2*xDotRel)/r2D^4;

b = b*180/pi;

== matlab function SC228_TrackedASModelUnitTest/SC-228 Sensor Model: Active Surveillance (Tracked)/Determine Track Validity/Compute Elevation/Compute elevation ==
  data: own_N_ft input; el_deg output; own_E_ft input; own_h_ft input; int_N_ft input; int_E_ft input; int_h_ft input; psi input; theta input; phi input
function el_deg = fcn(own_N_ft, own_E_ft, own_h_ft, int_N_ft, int_E_ft, int_h_ft, psi, theta, phi)
%#codegen
Ri = [int_N_ft-own_N_ft; int_E_ft-own_E_ft; -(int_h_ft-own_h_ft)];

ct   = cos(-theta);
st   = sin(-theta);
cphi = cos(phi); %1;%
sphi = sin(phi); %0;%
cpsi = cos(psi);
spsi = sin(psi);

M = [ ct*cpsi                  ct*spsi                     -st; ...
      sphi*st*cpsi-cphi*spsi   sphi*st*spsi+cphi*cpsi      sphi*ct; ...
      cphi*st*cpsi+sphi*spsi   cphi*st*spsi-sphi*cpsi      cphi*ct ];
  
Rb = M*Ri;

R = sqrt( Ri(1)^2+Ri(2)^2+Ri(3)^2 );
el = asin( Rb(3)/R );
el_deg = el*180/pi;

% roll = phi_deg;
% pitch = theta_deg;
% heading = psi_deg;
% 
% Ri = [int_N_ft-own_N_ft; int_E_ft-own_E_ft; -(int_h_ft-own_h_ft)];
% 
% Mroll = [1, 0, 0;...
%     0, cos(roll), sin(roll);...
%     0, -sin(roll), cos(roll)];
% 
% Mpitch = [cos(pitch), 0, -sin(pitch);...
%     0, 1, 0;...
%     sin(pitch), 0, cos(pitch)];
% 
% Mhead = [cos(heading), sin(heading), 0;...
%     -sin(heading), cos(heading), 0;...
%     0, 0, 1];
% 
% Mi2b = Mroll*Mpitch*Mhead; % inertial to body
%   
% Rb = Mi2b*Ri;
% 
% %R = sqrt( Ri(1)^2+Ri(2)^2+Ri(3)^2 );
% %az = atan2( Rb(2), Rb(1) );
% el = atan( -Rb(3)/sqrt(Ri(1)^2+Ri(2)^2) );
% 
% el_deg = el*180/pi;

end

== matlab function SC228_TrackedASModelUnitTest/SC-228 Sensor Model: Active Surveillance (Tracked)/Determine Track Validity/Determine Validity /MATLAB Function ==
  data: detectRange_ft input; isValid output; bearing_deg input; frontMaxRange_ft input; sideMaxRange_ft input; backMaxRange_ft input
function isValid = fcn(detectRange_ft, bearing_deg, frontMaxRange_ft, sideMaxRange_ft, backMaxRange_ft)
isValid = false;

%Need to wrap bearing_deg to 180
if bearing_deg >=180
    bearing_deg = bearing_deg - 2*180;
elseif bearing_deg <-180
    bearing_deg = bearing_deg + 2*180;
end

%#codegen
if(bearing_deg>=-45 && bearing_deg <=45) %front
    isValid = detectRange_ft<frontMaxRange_ft;
    
elseif (bearing_deg>=-135 && bearing_deg <=-45) || (bearing_deg>=45 && bearing_deg <=135) %side
    isValid = detectRange_ft<sideMaxRange_ft;
    
elseif (bearing_deg>=-180 && bearing_deg <=-135) || (bearing_deg>=135 && bearing_deg <=180) %back
    isValid = detectRange_ft<backMaxRange_ft;
    
end

== matlab function SC228_TrackedASModelUnitTest/SC-228 Sensor Model: Active Surveillance (Tracked)/Should provide an update if valid in any of the previous 10 deciseconds. ==
  data: isValid_out output; isValid input; prevValidHistory input; validHistory output
function [isValid_out, validHistory] = determineValidity(isValid, prevValidHistory)
%#codegen
validHistory = [isValid, prevValidHistory(1:9)];

isValid_out = max(validHistory);

== matlab function SC228_TrackedASModelUnitTest/cyl2xyz ==
  data: x output; r input; y output; rDot input; b input; bDot input; h input; hDot input; ownPsi input; ownPsiDot input; z output; xDot output; yDot output; zDot output; J output; K output
function [x,y,z,xDot,yDot,zDot,J,K] = fcn(r,rDot,b,bDot,h,hDot,ownPsi,ownPsiDot)
%#codegen
% Convert position and velocity of intruder relative to ownship from 
% range/bearing/altitude coordinates to North-East-Down coordinates. Also
% returns Jacobian blocks J and K, where 6x6 Jacobian = [J zeros; K J]

% because of independent noise, it's possible that estimated range can be
% smaller than estimated altitude --  in that case, use a range just
% slightly larger than the altitude
if abs(r) < abs(h)
    if r==0
        r = abs(h)+1;
    else
        r = sign(r)*abs(h)+1;
    end
end

r2D = sqrt(r^2 - h^2);

x = r2D*cos(b+ownPsi);
y = r2D*sin(b+ownPsi);
z = -h;

xDot = (1/r2D)*((r*rDot - h*hDot)*cos(b + ownPsi) - r2D*sin(b + ownPsi)*(bDot + ownPsiDot));
yDot = (1/r2D)*((r*rDot - h*hDot)*sin(b + ownPsi) + r2D*cos(b + ownPsi)*(bDot + ownPsiDot));
zDot = -hDot;

% Jacobian elements (for xyz -> cyl)

J = [  x/r   y/r    z/r ;
     -y/r2D^2  x/r2D^2   0  ;
          0       0 -1 ];
      
K = zeros(3,3);
K(1,1) = xDot/r - x*rDot/r^2;
K(1,2) = yDot/r - y*rDot/r^2;
K(1,3) = zDot/r - z*rDot/r^2;
K(2,1) = (yDot*y^2 + 2*x*xDot*y - yDot*x^2)/r2D^4;
K(2,2) = (xDot*y^2 - 2*x*y*yDot - x^2*xDot)/r2D^4;

% use Schur complement for cyl -> xyz
if ~isnan(rcond(J))
  J = inv(J);
  K = -J*K*J;
else
  J = nan(3);
  K = nan(3);
end
